simulink model "openloop"  (R2025b)
settings: Solver=ode3  StartTime=0.0  StopTime=1.5  FixedStep=1e-5  MaxStep=1e-5  RelTol=1e-3
values from neighbouring files (symbols this model uses):
  C = 470*10^-6    (= 0.00047)    [plotting.m]    (also in robusnost_grafici.m)
  L = 15.91*10^-3    (= 0.01591)    [plotting.m]    (also in robusnost_grafici.m = 0.012728)
  R = 52    [plotting.m]    (also in robusnost_grafici.m)
  sig2 = (0.02*x2e)^2    (= 0.2025)    [plotting.m]    (also in robusnost_grafici.m = 0)
  ue = 0.65217    [plotting.m]    (also in robusnost_grafici.m)
settings Model: Creator=User  LastModifiedBy=User

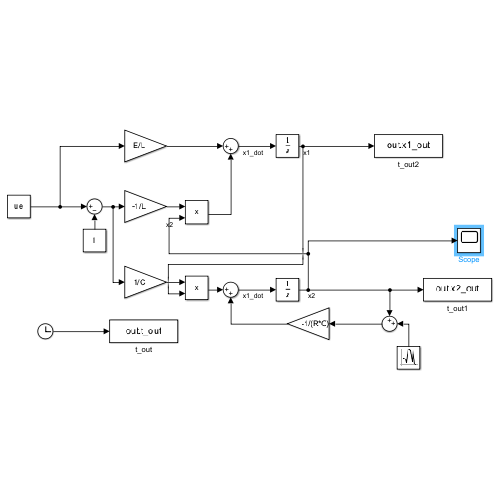
[thumbnail: Simulink's stored preview of the top-level diagram]
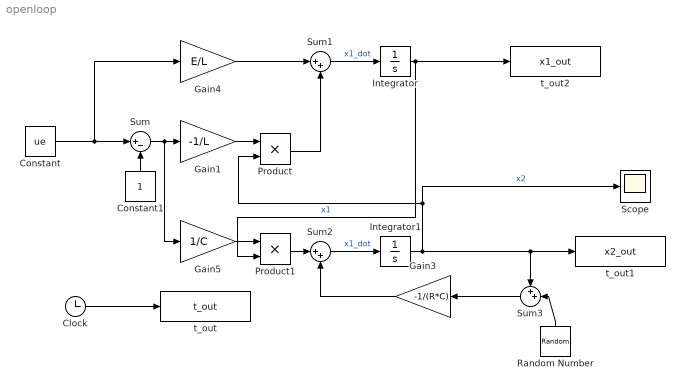
== system openloop ==
  Clock : Clock
  Constant : Constant  Value=ue
  Constant1 : Constant
  Gain1 : Gain  Gain=-1/L
  Gain3 : Gain  Gain=-1/(R*C)
  Gain4 : Gain  Gain=E/L
  Gain5 : Gain  Gain=1/C
  Integrator : Integrator
  Integrator1 : Integrator
  Product : Product
  Product1 : Product
  Random Number : RandomNumber  Variance=sig2  SampleTime=1e-5
  Scope : Scope
      settings: ActiveDisplayYMinimum=-23.8133994232757  ActiveDisplayYMaximum=-22.110951891793434
  Sum : Sum  Inputs=|+-
  Sum1 : Sum  Inputs=|++
  Sum2 : Sum  Inputs=|++
  Sum3 : Sum  Inputs=++|
  t_out : ToWorkspace  VariableName=t_out  SampleTime=-1
  t_out1 : ToWorkspace  VariableName=x2_out  SampleTime=-1
  t_out2 : ToWorkspace  VariableName=x1_out  SampleTime=-1
  wires:
  Product/1 -> Sum1/2
  Constant/1 -> Gain4/1, Sum/1
  Constant1/1 -> Sum/2
  Sum/1 -> Gain5/1, Gain1/1
  Gain1/1 -> Product/1
  Integrator1/1 -> Sum3/1, t_out1/1, Product/2, Scope/1  "x2"
  Sum1/1 -> Integrator/1  "x1_dot"
  Integrator/1 -> Product1/2, t_out2/1  "x1"
  Product1/1 -> Sum2/1
  Gain3/1 -> Sum2/2
  Sum2/1 -> Integrator1/1  "x1_dot"
  Clock/1 -> t_out/1
  Gain4/1 -> Sum1/1
  Gain5/1 -> Product1/1
  Random Number/1 -> Sum3/2
  Sum3/1 -> Gain3/1
